simulink model "Regler_LQR_GainSch"  (R2026a)
settings: Solver=ode23s  StartTime=tSim(1)  StopTime=tSim(end)  FixedStep=tStep  EnableMultiTasking=on
values from neighbouring files (symbols this model uses):
  A = [ 0,      1, 0,      0 ... (first row only)    [A4_4.m]    (also in reglerInit.m = [0, 1, 0, 0; reglerInit_fin.m = [0, 1, 0, 0; reglerInit_opt.m = [0, 1, 0, 0; reglerInit_opt1.m = [0, 1, 0, 0)
  A_obs = A - L_obs*C    [reglerInit.m]    (also in reglerInit_opt.m)
  B = [0; -30.49; 0; 30.49]    [A4_4.m]    (also in reglerInit.m; reglerInit_fin.m; reglerInit_gain_scheduling.m; reglerInit_opt.m)
  B_obs = [B, L_obs]    [reglerInit.m]    (also in reglerInit_opt.m)
  C = [1 0 0 0 ... (first row only)    [reglerInit.m]    (also in reglerInit_fin.m; reglerInit_gain_scheduling.m; reglerInit_opt.m; reglerInit_opt1.m)
  C_obs = eye(4)    [reglerInit.m]    (also in reglerInit_opt.m)
  D_obs = zeros(4,3)    [reglerInit.m]    (also in reglerInit_opt.m)
  K_lqi_noI = K_lqi    [reglerInit.m]
  K_schedule = zeros(n_mass, 5)    [reglerInit_gain_scheduling.m]
  lim_Pos = 2.45    [reglerInit.m]    (also in reglerInit_fin.m; reglerInit_gain_scheduling.m; reglerInit_opt.m; reglerInit_opt1.m)
  lim_rate = 1.3    [reglerInit.m]    (also in reglerInit_fin.m; reglerInit_gain_scheduling.m; reglerInit_opt.m; reglerInit_opt1.m)
  Lobs_schedule = zeros(n_mass, 8)    [reglerInit_gain_scheduling.m]
  mass_grid = 1:0.25:5    [reglerInit_gain_scheduling.m]
  xhat0 = [0, 0, 0, 0]    [reglerInit.m]    (also in reglerInit_fin.m = [0; 0; 0; 0]; reglerInit_gain_scheduling.m = [0; 0; 0; 0]; reglerInit_opt.m = [0; 0; 0; 0]; reglerInit_opt1.m = [0; 0; 0; 0])
undefined symbols (not defined in the file or in its folder): L
settings Model: Creator=Henning Schlüter  LastModifiedBy=louis
settings DataIOCC: SignalLoggingSaveFormat=ModelDataLogs
settings DebuggingCC: UnderspecifiedInitializationDetection=Classic  PregeneratedLibrarySubsystemCodeDiagnostic=none
settings HardwareCC: ProdHWDeviceType=32-bit Generic
settings GRTTargetCC: CombineOutputUpdateFcns=off  GRTInterface=on

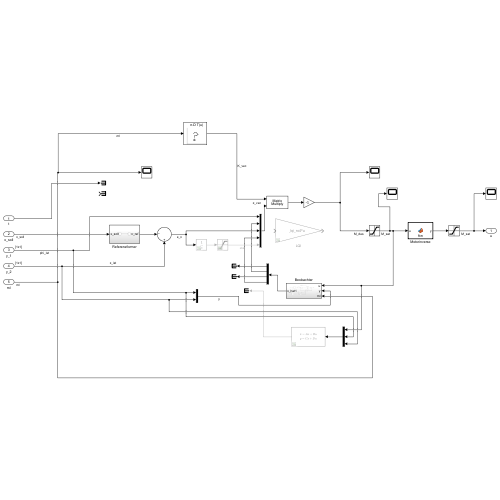
[thumbnail: Simulink's stored preview of the top-level diagram]
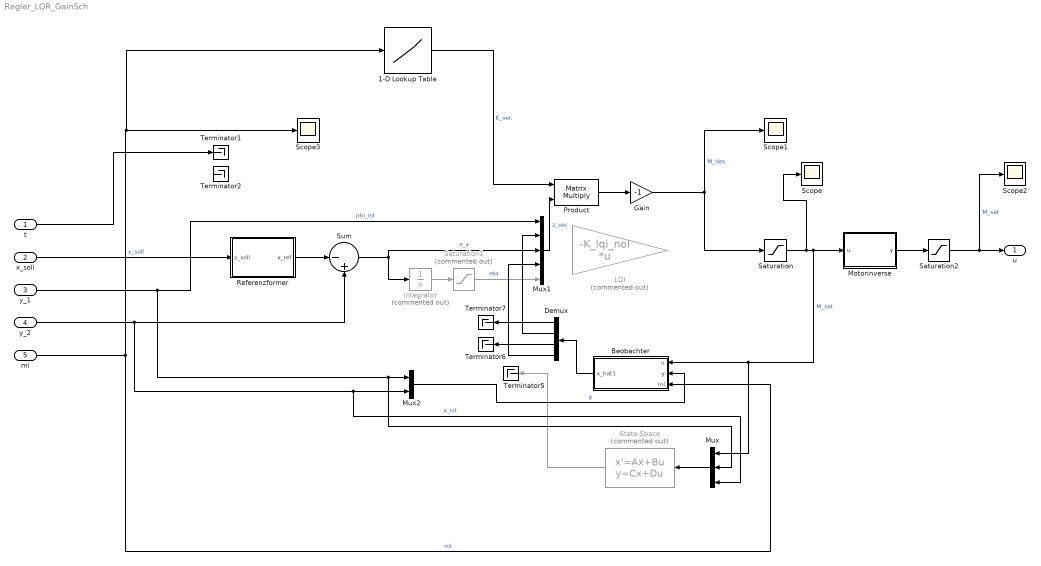
== system Regler_LQR_GainSch ==
  t : Inport  OutDataTypeStr=double  PortDimensions=1  SampleTime=0
  "x_soll " : Inport  Port=2  OutDataTypeStr=double  PortDimensions=1  SampleTime=0
  y_1 : Inport  Port=3  OutDataTypeStr=double  PortDimensions=[1 1]  SampleTime=0
  y_2 : Inport  Port=4  OutDataTypeStr=double  PortDimensions=[1 1]  SampleTime=0
  ml : Inport  Port=5  OutDataTypeStr=double  PortDimensions=1  SampleTime=0
  1-D Lookup Table : Lookup_n-D  NumberOfTableDimensions=1  BreakpointsForDimension1=mass_grid  Table=K_schedule  InternalRulePriority=Speed  RndMeth=Simplest
  Beobachter : Subsystem
  Demux : Demux
  Gain : Gain  Gain=-1
  Integrator : Integrator  Commented=on
  LQI : Gain  Commented=on  Gain=-K_lqi_noI  Multiplication=Matrix(K*u)
  Motorinverse : MATLAB Function  TreatAsAtomicUnit=on
  Mux : Mux  Inputs=3
  Mux1 : Mux  Inputs=5
  Mux2 : Mux  Inputs=2
  Product : Product  Multiplication=Matrix(*)
  Referenzformer : Subsystem
  Saturation : Saturate  UpperLimit=0.4  LowerLimit=-0.4
  Saturation1 : Saturate  Commented=on  UpperLimit=1  LowerLimit=-1
  Saturation2 : Saturate  UpperLimit=100  LowerLimit=-100
  Scope{,1..3} (4 alike) : Scope
      Scope settings: ActiveDisplayYMinimum=-0.324965965962021  ActiveDisplayYMaximum=0.5094991629225013
      Scope1 settings: ActiveDisplayYMinimum=-0.094687281937852363  ActiveDisplayYMaximum=1.6990664417619266
      Scope2 settings: ActiveDisplayYMinimum=94.50632842581112  ActiveDisplayYMaximum=100.54238579484297  DataLoggingVariableName=ScopeData2
      Scope3 settings: ActiveDisplayYMinimum=0.60192793931732025  ActiveDisplayYMaximum=5.3638327012220817  DataLoggingVariableName=ScopeData3
  State-Space : StateSpace  Commented=on  A=A_obs  B=B_obs  C=C_obs  D=D_obs  InitialCondition=0
  Sum : Sum  Inputs=|-+
  Terminator{1..2,5..7} (5 alike) : Terminator
  u : Outport  OutDataTypeStr=double  PortDimensions=1  VectorParamsAs1DForOutWhenUnconnected=off
  wires:
  Saturation/1 -> Scope/1, Motorinverse/1(u), Beobachter/1(u), Mux/1  "M_sat"
  Saturation1/1 -> Mux1/5  "eta"
  Demux/3 -> Terminator6/1
  Integrator/1 -> Saturation1/1
  Demux/4 -> Mux1/4
  Motorinverse/1(y) -> Saturation2/1
  Demux/1 -> Terminator7/1
  State-Space/1 -> Terminator5/1
  Referenzformer/1(x_ref) -> Sum/1
  Demux/2 -> Mux1/2
  y_2/1 -> Mux/3, Mux2/2, Sum/2  "x_ist"
  Saturation2/1 -> u/1, Scope2/1  "M_sat"
  Beobachter/1(x_hat1) -> Demux/1
  Mux/1 -> State-Space/1
  t/1 -> Terminator1/1
  Gain/1 -> Saturation/1, Scope1/1  "M_des"
  Mux2/1 -> Beobachter/2(y)  "y"
  "x_soll "/1 -> Referenzformer/1(x_soll)  "x_soll"
  Sum/1 -> Mux1/3, Integrator/1  "e_x"
  y_1/1 -> Mux1/1, Mux/2, Mux2/1  "phi_ist"
  1-D Lookup Table/1 -> Product/1  "K_vec"
  ml/1 -> Beobachter/3(ml), 1-D Lookup Table/1, Scope3/1  "ml"
  Mux1/1 -> Product/2  "z_vec"
  Product/1 -> Gain/1

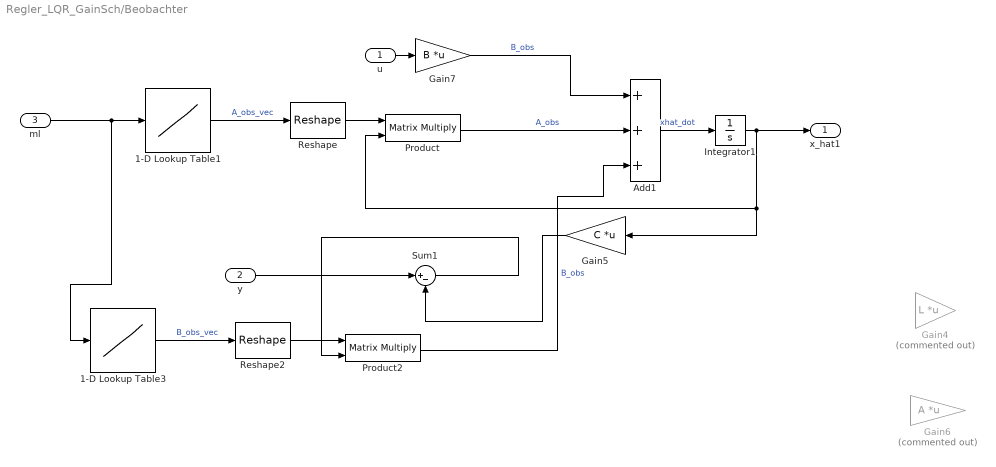
== system Regler_LQR_GainSch/Beobachter ==
  u : Inport
  y : Inport  Port=2
  ml : Inport  Port=3
  1-D Lookup Table1 : Lookup_n-D  NumberOfTableDimensions=1  BreakpointsForDimension1=mass_grid  Table=A_obs  InternalRulePriority=Speed  RndMeth=Simplest
  1-D Lookup Table3 : Lookup_n-D  NumberOfTableDimensions=1  BreakpointsForDimension1=mass_grid  Table=Lobs_schedule  InternalRulePriority=Speed  RndMeth=Simplest
  Add1 : Sum  Inputs=+++
  Gain4 : Gain  Commented=on  Gain=L  Multiplication=Matrix(K*u)
  Gain5 : Gain  Gain=C  Multiplication=Matrix(K*u)
  Gain6 : Gain  Commented=on  Gain=A  Multiplication=Matrix(K*u)
  Gain7 : Gain  Gain=B  Multiplication=Matrix(K*u)
  Integrator1 : Integrator  InitialCondition=xhat0
  Product : Product  Multiplication=Matrix(*)
  Product2 : Product  Multiplication=Matrix(*)
  Reshape : Reshape  OutputDimensionality=Customize  OutputDimensions=[4,4]
  Reshape2 : Reshape  OutputDimensionality=Customize  OutputDimensions=[4,2]
  Sum1 : Sum  Inputs=|+-
  x_hat1 : Outport
  wires:
  u/1 -> Gain7/1
  Product/1 -> Add1/2  "A_obs"
  Sum1/1 -> Product2/2
  Gain7/1 -> Add1/1  "B_obs"
  Reshape/1 -> Product/1
  ml/1 -> 1-D Lookup Table3/1, 1-D Lookup Table1/1
  1-D Lookup Table3/1 -> Reshape2/1  "B_obs_vec"
  Reshape2/1 -> Product2/1
  1-D Lookup Table1/1 -> Reshape/1  "A_obs_vec"
  Add1/1 -> Integrator1/1  "xhat_dot"
  y/1 -> Sum1/1
  Integrator1/1 -> Gain5/1, Product/2, x_hat1/1
  Gain5/1 -> Sum1/2
  Product2/1 -> Add1/3  "B_obs"

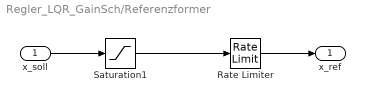
== system Regler_LQR_GainSch/Referenzformer ==
  x_soll : Inport
  Rate Limiter : RateLimiter  RisingSlewLimit=lim_rate  FallingSlewLimit=-lim_rate  SampleTimeMode=inherited
  Saturation1 : Saturate  UpperLimit=lim_Pos  LowerLimit=-lim_Pos
  x_ref : Outport
  wires:
  Rate Limiter/1 -> x_ref/1
  x_soll/1 -> Saturation1/1
  Saturation1/1 -> Rate Limiter/1

== matlab function Regler_LQR_GainSch/Motorinverse ==
  data: u input; y output
function y = fcn(u)

y = sign(u(1)/2)*(9.434*abs(u(1)/2))^2*100/3.56;
